simulink model "HW2"  (R2024b)
settings: Solver=VariableStepAuto  StartTime=0.0  StopTime=10.0  RelTol=1e-3
settings Model: Creator=iremm  LastModifiedBy=iremm

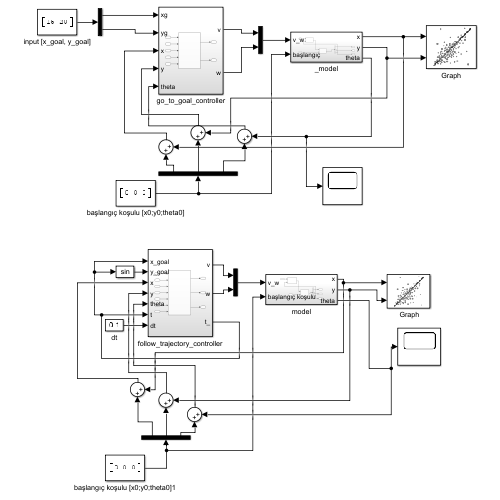
[thumbnail: Simulink's stored preview of the top-level diagram]
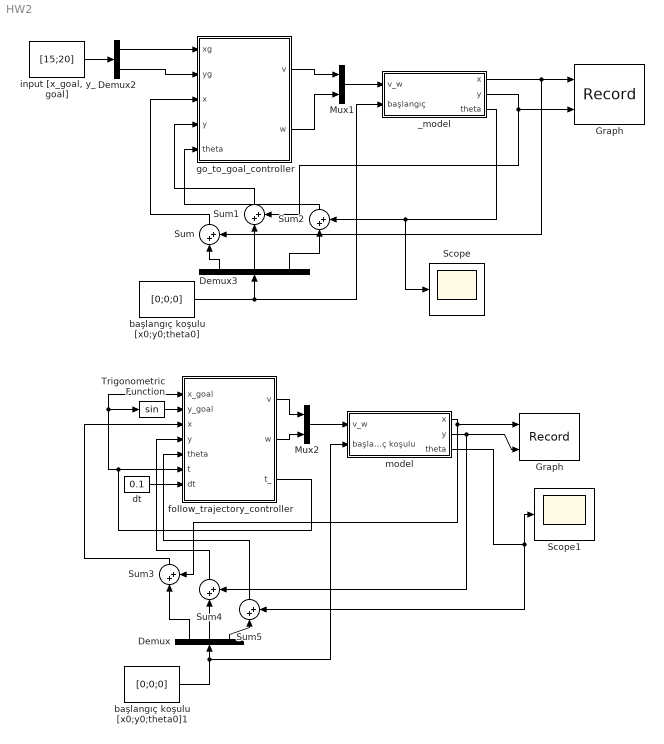
== system HW2 ==
  " Graph" : Record  FileSettingsInternal="{\"entries\":[{\"content\":{\"excelSettings\":{\"content\":{},\"type\":\"Streamout.ExcelSettings\"}},\"type\":\"Streamout.FileSettingStorage\",\"uuid\":\"\"}],\"packageUris\":[\"http:\\/\\/schema.mathworks.com\\/mf0\\/streamout_blocks\\/R2020a\"],\"version\":\"1.0\"}"  Layout=[1 1]  SignalsInternal="{\"entries\":[{\"content\":{\"signals\":[{\"content\":{\"blockPath\":[],\"dimensions\":[1],\"domain\":\"\",\"lineColor\":\"#a2142f\",\"plots\":[ 1 ],\"port\":1,\"signalID\":1,\"signalName\":\"XY Graph:1\"},\"type\":\"RecordBlkView.Signal\",\"uuid\":\"\"},{\"content\":{\"blockPath\":[],\"dimensions\":[1],\"domain\":\"\",\"lineColor\":\"#139fff\",\"plots\":[ 1 ],\"port\":2,\"signalID\":2,\"signalName\":\"XY Graph:2\"},\"type\":\"RecordBlkView.Signal\",\"uuid\":\"\"}]},\"type\":\"RecordBlkView.InputSignals\",\"uuid\":\"\"}],\"packageUris\":[\"http:\\/\\/schema.mathworks.com\\/mf0\\/streamout_blocks\\/R2020a\"],\"version\":\"1.0\"}"  VisualizationBindings="{\"xyplotplugin\":{\"info\":[{\"series\":[{\"bindingParametersList\":[{\"parameter\":\"X-Axis\",\"signalID\":1,\"signalName\":\"XY Graph:1\"},{\"parameter\":\"Y-Axis\",\"signalID\":2,\"signalName\":\"XY Graph:2\"}],\"seriesID\":0}],\"subplotID\":1}]}}"  CompatibilityTag=XY  st=-1
  Demux : Demux  Outputs=3
  Demux2 : Demux  Outputs=2
  Demux3 : Demux  Outputs=3
  Graph : Record  FileSettingsInternal="{\"entries\":[{\"content\":{\"excelSettings\":{\"content\":{},\"type\":\"Streamout.ExcelSettings\"}},\"type\":\"Streamout.FileSettingStorage\",\"uuid\":\"\"}],\"packageUris\":[\"http:\\/\\/schema.mathworks.com\\/mf0\\/streamout_blocks\\/R2020a\"],\"version\":\"1.0\"}"  Layout=[1 1]  SignalsInternal="{\"entries\":[{\"content\":{\"signals\":[{\"content\":{\"blockPath\":[],\"dimensions\":[1],\"domain\":\"\",\"lineColor\":\"#a2142f\",\"plots\":[ 1 ],\"port\":1,\"signalID\":1,\"signalName\":\"XY Graph:1\"},\"type\":\"RecordBlkView.Signal\",\"uuid\":\"\"},{\"content\":{\"blockPath\":[],\"dimensions\":[1],\"domain\":\"\",\"lineColor\":\"#139fff\",\"plots\":[ 1 ],\"port\":2,\"signalID\":2,\"signalName\":\"XY Graph:2\"},\"type\":\"RecordBlkView.Signal\",\"uuid\":\"\"}]},\"type\":\"RecordBlkView.InputSignals\",\"uuid\":\"\"}],\"packageUris\":[\"http:\\/\\/schema.mathworks.com\\/mf0\\/streamout_blocks\\/R2020a\"],\"version\":\"1.0\"}"  VisualizationBindings="{\"xyplotplugin\":{\"info\":[{\"series\":[{\"bindingParametersList\":[{\"parameter\":\"X-Axis\",\"signalID\":1,\"signalName\":\"XY Graph:1\"},{\"parameter\":\"Y-Axis\",\"signalID\":2,\"signalName\":\"XY Graph:2\"}],\"seriesID\":0}],\"subplotID\":1}]}}"  CompatibilityTag=XY  st=-1
  Mux1 : Mux  Inputs=2
  Mux2 : Mux  Inputs=2
  Scope : Scope
  Scope1 : Scope
  Sum{,1..5} (6 alike) : Sum  Inputs=|++
  Trigonometric Function : Trigonometry
  _model : Subsystem
  başlangıç koşulu [x0;y0;theta0] : Constant  Value=[0;0;0]
  başlangıç koşulu [x0;y0;theta0]1 : Constant  Value=[0;0;0]
  dt : Constant  Value=0.1
  follow_trajectory_controller : Subsystem
  go_to_goal_controller : Subsystem
  "input [x_goal, y_goal]" : Constant  Value=[15;20]
  model : Subsystem
  wires:
  go_to_goal_controller/1(v) -> Mux1/1
  başlangıç koşulu [x0;y0;theta0]/1 -> _model/2(başlangıç), Demux3/1
  _model/2(y) -> Sum1/2, Graph/2
  Sum1/1 -> go_to_goal_controller/4(y)
  go_to_goal_controller/2(w) -> Mux1/2
  Demux3/3 -> Sum2/1
  Demux3/2 -> Sum1/1
  Demux2/2 -> go_to_goal_controller/2(yg)
  "input [x_goal, y_goal]"/1 -> Demux2/1
  Demux3/1 -> Sum/1
  Sum2/1 -> go_to_goal_controller/5(theta)
  Demux2/1 -> go_to_goal_controller/1(xg)
  _model/1(x) -> Sum/2, Graph/1
  Sum/1 -> go_to_goal_controller/3(x)
  _model/3(theta) -> Scope/1, Sum2/2
  Mux1/1 -> _model/1(v_w)
  Demux/1 -> Sum3/1
  Trigonometric Function/1 -> follow_trajectory_controller/2(y_goal)
  Sum3/1 -> follow_trajectory_controller/3(x)
  model/1(x) -> " Graph"/1, Sum3/2
  Demux/2 -> Sum4/1
  follow_trajectory_controller/2(w) -> Mux2/2
  Demux/3 -> Sum5/1
  Sum5/1 -> follow_trajectory_controller/5(theta)
  model/2(y) -> Sum4/2, " Graph"/2
  dt/1 -> follow_trajectory_controller/7(dt)
  Sum4/1 -> follow_trajectory_controller/4(y)
  Mux2/1 -> model/1(v_w)
  follow_trajectory_controller/3(t_) -> follow_trajectory_controller/6(t), follow_trajectory_controller/1(x_goal), Trigonometric Function/1
  model/3(theta) -> Sum5/2, Scope1/1
  follow_trajectory_controller/1(v) -> Mux2/1
  başlangıç koşulu [x0;y0;theta0]1/1 -> model/2(başlangıç koşulu), Demux/1

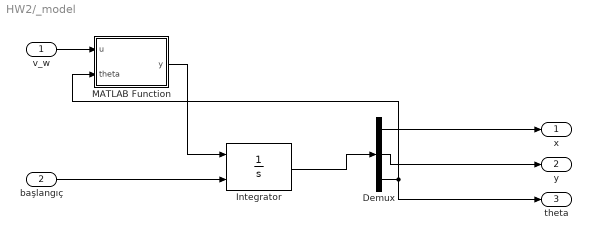
== system HW2/_model ==
  v_w : Inport
  başlangıç : Inport  Port=2
  Demux : Demux  Outputs=3
  Integrator : Integrator  InitialConditionSource=external
  MATLAB Function : MATLAB Function  TreatAsAtomicUnit=on
  x : Outport
  y : Outport  Port=2
  theta : Outport  Port=3
  wires:
  MATLAB Function/1(y) -> Integrator/1
  Demux/3 -> theta/1, MATLAB Function/2(theta)
  Integrator/1 -> Demux/1
  Demux/1 -> x/1
  başlangıç/1 -> Integrator/2
  v_w/1 -> MATLAB Function/1(u)
  Demux/2 -> y/1

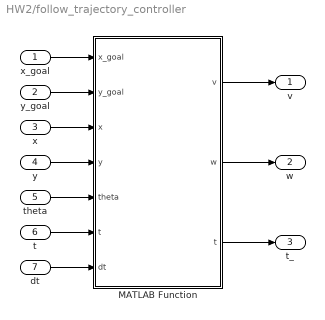
== system HW2/follow_trajectory_controller ==
  x_goal : Inport
  y_goal : Inport  Port=2
  x : Inport  Port=3
  y : Inport  Port=4
  theta : Inport  Port=5
  t : Inport  Port=6
  dt : Inport  Port=7
  MATLAB Function : MATLAB Function  TreatAsAtomicUnit=on
  v : Outport
  w : Outport  Port=2
  t_ : Outport  Port=3
  wires:
  MATLAB Function/1(v) -> v/1
  MATLAB Function/2(w) -> w/1
  x_goal/1 -> MATLAB Function/1(x_goal)
  y_goal/1 -> MATLAB Function/2(y_goal)
  x/1 -> MATLAB Function/3(x)
  y/1 -> MATLAB Function/4(y)
  theta/1 -> MATLAB Function/5(theta)
  t/1 -> MATLAB Function/6("t ")
  dt/1 -> MATLAB Function/7(dt)
  MATLAB Function/3(t) -> t_/1

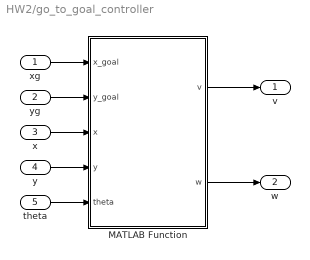
== system HW2/go_to_goal_controller ==
  xg : Inport
  yg : Inport  Port=2
  x : Inport  Port=3
  y : Inport  Port=4
  theta : Inport  Port=5
  MATLAB Function : MATLAB Function  TreatAsAtomicUnit=on
  v : Outport
  w : Outport  Port=2
  wires:
  theta/1 -> MATLAB Function/5(theta)
  y/1 -> MATLAB Function/4(y)
  x/1 -> MATLAB Function/3(x)
  yg/1 -> MATLAB Function/2(y_goal)
  xg/1 -> MATLAB Function/1(x_goal)
  MATLAB Function/1(v) -> v/1
  MATLAB Function/2(w) -> w/1

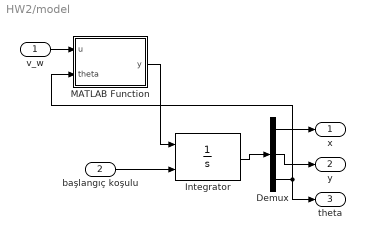
== system HW2/model ==
  v_w : Inport
  başlangıç koşulu : Inport  Port=2
  Demux : Demux  Outputs=3
  Integrator : Integrator  InitialConditionSource=external
  MATLAB Function : MATLAB Function  TreatAsAtomicUnit=on
  x : Outport
  y : Outport  Port=2
  theta : Outport  Port=3
  wires:
  MATLAB Function/1(y) -> Integrator/1
  Demux/3 -> theta/1, MATLAB Function/2(theta)
  Integrator/1 -> Demux/1
  Demux/1 -> x/1
  başlangıç koşulu/1 -> Integrator/2
  v_w/1 -> MATLAB Function/1(u)
  Demux/2 -> y/1

== matlab function HW2/go_to_goal_controller/MATLAB Function ==
  data: x_goal input; y_goal input; x input; y input; v output; theta input; w output
function [v,w]= fcn(x_goal,y_goal,x,y,theta)
Kv = 1.0;
Kh = 1.0;
delta_x = x_goal - x;
delta_y = y_goal - y;
theta_g = atan2(delta_y, delta_x);
delta_theta = theta_g - theta;
delta_theta = atan2(sin(delta_theta), cos(delta_theta));
distance = sqrt(delta_x^2 + delta_y^2);
vt = Kv * distance;
wt = Kh * delta_theta;

if vt > 1
    vt = 1;
end
if wt > pi/4
    wt = pi/4;
end

v = vt;
w = wt;

== matlab function HW2/follow_trajectory_controller/MATLAB Function ==
  data: x_goal input; y_goal input; x input; y input; v output; theta input; w output; t input; dt input; t output
function [v,w,t]= fcn(x_goal, y_goal, x, y, theta,t ,dt)

Kv = 1.0;
Ki = 1.0;
Kh = 1.0;
t = t + dt;
x_g = x_goal;
y_g = y_goal;
e = sqrt((x_g - x)^2 + (y_g - y)^2) - d;
vt = Kv * e + Ki * (e*t - e*(t-dt));
theta_g = atan2(y_g - y, x_g - x);
wt = Kh * (atan2(sin(theta_g - theta), cos(theta_g - theta)));
v = vt;
w = wt;

== matlab function HW2/model/MATLAB Function ==
  data: u input; y output; theta input
function y = fcn(u, theta)

v = u(1);
w = u(2);

y = [v*cos(theta); v*sin(theta); w];

== matlab function HW2/_model/MATLAB Function ==
  data: u input; y output; theta input
function y = fcn(u, theta)
v = u(1);
w = u(2);
y = [v*cos(theta); v*sin(theta); w];
